simulink model "simulink_model"  (R2025b)
settings: Solver=VariableStepAuto  StartTime=0.0  StopTime=10  MaxStep=0.01  RelTol=1e-3
InitFcn:
  | addpath('C:\Users\prest\Documents\GitHub\NUSTARS\Roll-Control\Plotting');
  | % Define the directory containing the CSV files
  | data_dir = 'C:\Users\prest\Documents\GitHub\NUSTARS\Roll-Control\Plotting\Data';
  | addpath('C:\Users\prest\Documents\GitHub\NUSTARS\Roll-Control\Plotting');
  | 
  | % Get a list of all CSV files in the directory
  | csv_files = dir(fullfile(data_dir, '*.csv'));
  | 
  | for k = 1:length(csv_files)
  |     flight_csv = fullfile(data_dir, csv_files(k).name);
  |     ft_main_roll_only(flight_csv);
  | end
libraries: slpidlib x2
settings Model: Creator=maxhu  LastModifiedBy=prest

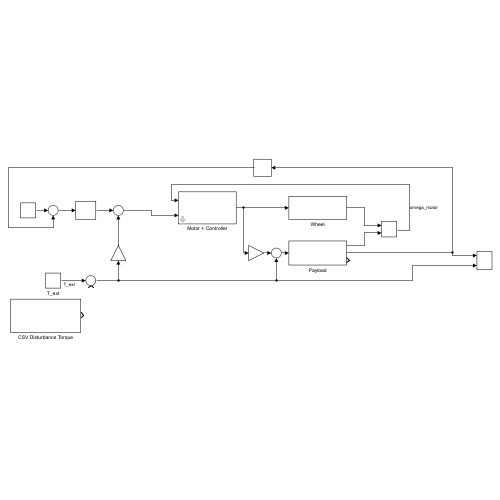
[thumbnail: Simulink's stored preview of the top-level diagram]
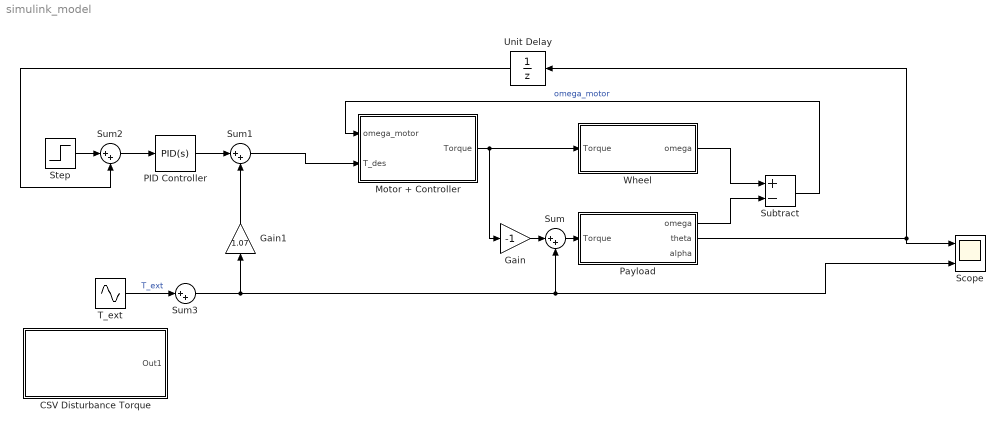
== system simulink_model ==
  CSV Disturbance Torque : Subsystem
  Gain : Gain  Gain=-1
  Gain1 : Gain  Gain=1.07
  Motor + Controller : Subsystem  mask{V_supply=12, T_max=1.65}
      mask prompts: V_supply "Battery Voltage [V]"; T_max "Max Torque [N*m]"
  PID Controller : slpidlib/PID Controller  Controller=PID  Form=Parallel  TimeDomain=Continuous-time  UseExternalTs=off  SampleTime=-1  IntegratorMethod=Forward Euler  FilterMethod=Forward Euler  ControllerParametersSource=internal  P=2e-1  I=5e-2  UseKiTs=off  D=8e-2  UseExternalDerivativeSource=off  N=30  UseFilter=on  TunerSelectOption=Transfer Function Based (PID Tuner App)  InitialConditionSource=internal  InitialConditionForIntegrator=0  InitialConditionForFilter=0  DifferentiatorICPrevScaledInput=0  ExternalReset=none  TrackingMode=off  Kt=1  LimitOutput=off  SatLimitsSource=internal  UpperSaturationLimit=inf  LowerSaturationLimit=-inf  LinearizeAsGain=on  AntiWindupMode=none  Kb=1  LimitIntegrator=on  UpperIntegratorSaturationLimit=1  LowerIntegratorSaturationLimit=-1  POutMin=[]  POutMax=[]  IOutMin=[]  IOutMax=[]  DOutMin=[]  DOutMax=[]  NOutMin=[]  NOutMax=[]  SumOutMin=[]  SumOutMax=[]  SaturationOutMin=[]  SaturationOutMax=[]  PParamMin=[]  PParamMax=[]  IParamMin=[]  IParamMax=[]  DParamMin=[]  DParamMax=[]  NParamMin=[]  NParamMax=[]  KbParamMin=[]  KbParamMax=[]  KtParamMin=[]  KtParamMax=[]  KbOutMin=[]  KbOutMax=[]  KtOutMin=[]  KtOutMax=[]  IntegratorOutMin=[]  IntegratorOutMax=[]  FilterOutMin=[]  FilterOutMax=[]  SumI1OutMin=[]  SumI1OutMax=[]  SumI2OutMin=[]  SumI2OutMax=[]  SumI3OutMin=[]  SumI3OutMax=[]  SumI4OutMin=[]  SumI4OutMax=[]  SumDOutMin=[]  SumDOutMax=[]  DifferentiatorOutMin=[]  DifferentiatorOutMax=[]  FilterDiffOutCoefMin=[]  FilterDiffOutCoefMax=[]  ReciprocalOutMin=[]  ReciprocalOutMax=[]  SumDenOutMin=[]  SumDenOutMax=[]  SumNumOutMin=[]  SumNumOutMax=[]  DivideOutMin=[]  DivideOutMax=[]  UdiffTsProdOutMin=[]  UdiffTsProdOutMax=[]  NTsProdOutMin=[]  NTsProdOutMax=[]  UintegralTsProdOutMin=[]  UintegralTsProdOutMax=[]  UngainTsProdOutMin=[]  UngainTsProdOutMax=[]  ClampingZeroOutDataTypeStr=Inherit: Inherit via back propagation  ClampingZeroOutMin=[]  ClampingZeroOutMax=[]  FilterDenConstantOutDataTypeStr=Inherit: Inherit via back propagation  FilterDenConstantOutMin=[]  FilterDenConstantOutMax=[]  PCopyOutDataTypeStr=Inherit: Inherit via back propagation  PCopyOutMin=[]  PCopyOutMax=[]  NCopyOutDataTypeStr=Inherit: Inherit via back propagation  NCopyOutMin=[]  NCopyOutMax=[]  IntegratorContinuousStateAttributes=''  IntegratorStateMustResolveToSignalObject=off  IntegratorRTWStateStorageClass=Auto  FilterContinuousStateAttributes=''  FilterStateMustResolveToSignalObject=off  FilterRTWStateStorageClass=Auto  ParallelPVariant=InternalParameters  IdealPVariant=Disabled  IVariant=InternalParameters  DVariant=InternalParameters  IntegratorVariant=Continuous  SatVariant=Disabled  AWVariant=Passthrough  PCopyVariant=Disabled  TRVariant=Disabled  FdbkBlocksVariant=Forward  IdealPFdbkVariant=Disabled  SatFdbkVariant=Disabled  DerivativeFilterVariant=ContFilter  NVariant=InternalParameters  NCopyVariant=Disabled  FilterICVariant=InternalICsFilter  IntegratorICVariant=InternalICs  ExternalResetVariant=Disabled  TRSumVariant=Passthrough  SumFdbkVariant=Disabled  SumVariant=Sum_PID  TsampFilterVariant=InternalTs  TsampNgainVariant=Passthrough  TsampIntegralVariant=Passthrough  ExternalSaturationOutDataTypeStr=Inherit: Same as second input  DerivativeSourceVariant=ErrorSignal  PreIntVariant=InternalPreInt
  Payload : Subsystem
  Scope : Scope  NumInputPorts=2
      settings: ActiveDisplayYMinimum=-2.4708061966220987  ActiveDisplayYMaximum=3.9877688102350177
  Step : Step  After=-1  SampleTime=0
  Subtract : Sum  Inputs=+-
  Sum{,1..3} (4 alike) : Sum  Inputs=|++
  T_ext : Sin  Frequency=7  SampleTime=0
  Unit Delay : UnitDelay  SampleTime=1e-3  HasFrameUpgradeWarning=on
  Wheel : Subsystem
  wires:
  Wheel/1(omega) -> Subtract/1
  Gain/1 -> Sum/1
  Sum/1 -> Payload/1(Torque)
  Payload/1(omega) -> Subtract/2
  Motor + Controller/1(Torque) -> Gain/1, Wheel/1(Torque)
  Subtract/1 -> Motor + Controller/1(omega_motor)  "omega_motor"
  Payload/2(theta) -> Scope/1, Unit Delay/1
  Step/1 -> Sum2/1
  Sum2/1 -> PID Controller/1
  Unit Delay/1 -> Sum2/2
  Sum1/1 -> Motor + Controller/2(T_des)
  Sum3/1 -> Scope/2, Sum/2, Gain1/1
  Gain1/1 -> Sum1/2
  PID Controller/1 -> Sum1/1
  T_ext/1 -> Sum3/1  "T_ext"

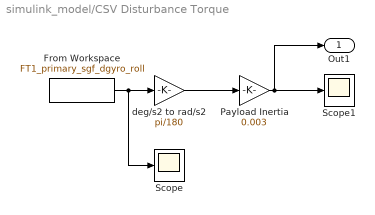
== system simulink_model/CSV Disturbance Torque ==
  From Workspace : FromWorkspace  VariableName=FT1_primary_sgf_dgyro_roll
  Payload Inertia : Gain  Gain=0.003
  Scope : Scope
      settings: ActiveDisplayYMinimum=-1  ActiveDisplayYMaximum=1  DataLoggingVariableName=ScopeData3
  Scope1 : Scope
      settings: ActiveDisplayYMinimum=-0.32143714141880175  ActiveDisplayYMaximum=0.6278113122409269
  deg/s2 to rad/s2 : Gain  Gain=pi/180
  Out1 : Outport
  wires:
  From Workspace/1 -> Scope/1, deg/s2 to rad/s2/1
  Payload Inertia/1 -> Out1/1, Scope1/1
  deg/s2 to rad/s2/1 -> Payload Inertia/1

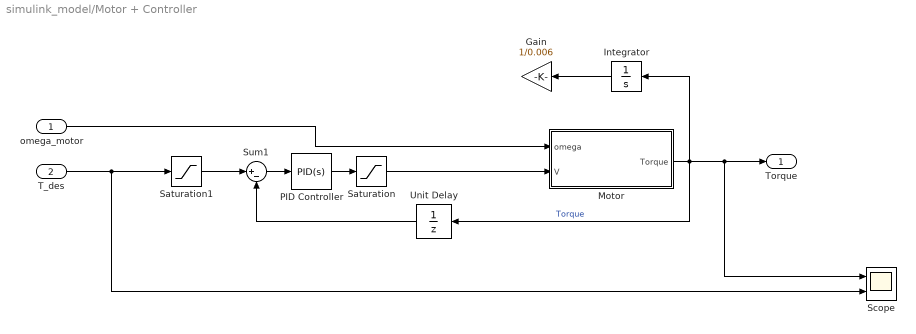
== system simulink_model/Motor + Controller ==
  omega_motor : Inport
  T_des : Inport  Port=2
  Gain : Gain  Gain=1/0.006
  Integrator : Integrator
  Motor : Subsystem  mask{w_nl=182, T_stall=10.9, L=0.000024}
      mask prompts: w_nl "No load speed [rad/s]"; T_stall "Stall torque [N*m]"; L "Inductance [H]"
  PID Controller : slpidlib/PID Controller  Controller=PID  Form=Parallel  TimeDomain=Continuous-time  UseExternalTs=off  SampleTime=-1  IntegratorMethod=Forward Euler  FilterMethod=Forward Euler  ControllerParametersSource=internal  P=1.24  I=650  UseKiTs=off  D=0.4e-4  UseExternalDerivativeSource=off  N=300  UseFilter=on  TunerSelectOption=Transfer Function Based (PID Tuner App)  InitialConditionSource=internal  InitialConditionForIntegrator=0  InitialConditionForFilter=0  DifferentiatorICPrevScaledInput=0  ExternalReset=none  TrackingMode=off  Kt=1  LimitOutput=on  SatLimitsSource=internal  UpperSaturationLimit=12  LowerSaturationLimit=-12  LinearizeAsGain=on  AntiWindupMode=none  Kb=1  LimitIntegrator=on  UpperIntegratorSaturationLimit=40  LowerIntegratorSaturationLimit=-40  POutMin=[]  POutMax=[]  IOutMin=[]  IOutMax=[]  DOutMin=[]  DOutMax=[]  NOutMin=[]  NOutMax=[]  SumOutMin=[]  SumOutMax=[]  SaturationOutMin=[]  SaturationOutMax=[]  PParamMin=[]  PParamMax=[]  IParamMin=[]  IParamMax=[]  DParamMin=[]  DParamMax=[]  NParamMin=[]  NParamMax=[]  KbParamMin=[]  KbParamMax=[]  KtParamMin=[]  KtParamMax=[]  KbOutMin=[]  KbOutMax=[]  KtOutMin=[]  KtOutMax=[]  IntegratorOutMin=[]  IntegratorOutMax=[]  FilterOutMin=[]  FilterOutMax=[]  SumI1OutMin=[]  SumI1OutMax=[]  SumI2OutMin=[]  SumI2OutMax=[]  SumI3OutMin=[]  SumI3OutMax=[]  SumI4OutMin=[]  SumI4OutMax=[]  SumDOutMin=[]  SumDOutMax=[]  DifferentiatorOutMin=[]  DifferentiatorOutMax=[]  FilterDiffOutCoefMin=[]  FilterDiffOutCoefMax=[]  ReciprocalOutMin=[]  ReciprocalOutMax=[]  SumDenOutMin=[]  SumDenOutMax=[]  SumNumOutMin=[]  SumNumOutMax=[]  DivideOutMin=[]  DivideOutMax=[]  UdiffTsProdOutMin=[]  UdiffTsProdOutMax=[]  NTsProdOutMin=[]  NTsProdOutMax=[]  UintegralTsProdOutMin=[]  UintegralTsProdOutMax=[]  UngainTsProdOutMin=[]  UngainTsProdOutMax=[]  ClampingZeroOutDataTypeStr=Inherit: Inherit via back propagation  ClampingZeroOutMin=[]  ClampingZeroOutMax=[]  FilterDenConstantOutDataTypeStr=Inherit: Inherit via back propagation  FilterDenConstantOutMin=[]  FilterDenConstantOutMax=[]  PCopyOutDataTypeStr=Inherit: Inherit via back propagation  PCopyOutMin=[]  PCopyOutMax=[]  NCopyOutDataTypeStr=Inherit: Inherit via back propagation  NCopyOutMin=[]  NCopyOutMax=[]  IntegratorContinuousStateAttributes=''  IntegratorStateMustResolveToSignalObject=off  IntegratorRTWStateStorageClass=Auto  FilterContinuousStateAttributes=''  FilterStateMustResolveToSignalObject=off  FilterRTWStateStorageClass=Auto  ParallelPVariant=InternalParameters  IdealPVariant=Disabled  IVariant=InternalParameters  DVariant=InternalParameters  IntegratorVariant=Continuous  SatVariant=Disabled  AWVariant=Passthrough  PCopyVariant=Disabled  TRVariant=Disabled  FdbkBlocksVariant=Forward  IdealPFdbkVariant=Disabled  SatFdbkVariant=Disabled  DerivativeFilterVariant=ContFilter  NVariant=InternalParameters  NCopyVariant=Disabled  FilterICVariant=InternalICsFilter  IntegratorICVariant=InternalICs  ExternalResetVariant=Disabled  TRSumVariant=Passthrough  SumFdbkVariant=Disabled  SumVariant=Sum_PID  TsampFilterVariant=InternalTs  TsampNgainVariant=Passthrough  TsampIntegralVariant=Passthrough  ExternalSaturationOutDataTypeStr=Inherit: Same as second input  DerivativeSourceVariant=ErrorSignal  PreIntVariant=InternalPreInt
  Saturation : Saturate  UpperLimit=V_supply  LowerLimit=-V_supply
  Saturation1 : Saturate  UpperLimit=T_max  LowerLimit=-T_max
  Scope : Scope  NumInputPorts=2
      settings: ActiveDisplayYMinimum=-1  ActiveDisplayYMaximum=1  DataLoggingVariableName=ScopeData2
  Sum1 : Sum  Inputs=|+-
  Unit Delay : UnitDelay  SampleTime=0.0005  HasFrameUpgradeWarning=on
  Torque : Outport
  wires:
  Sum1/1 -> PID Controller/1
  Unit Delay/1 -> Sum1/2
  Motor/1(Torque) -> Integrator/1, Unit Delay/1, Scope/1, Torque/1  "Torque"
  PID Controller/1 -> Saturation/1
  Integrator/1 -> Gain/1
  Saturation/1 -> Motor/2(V)
  Saturation1/1 -> Sum1/1
  T_des/1 -> Scope/2, Saturation1/1
  omega_motor/1 -> Motor/1(omega)

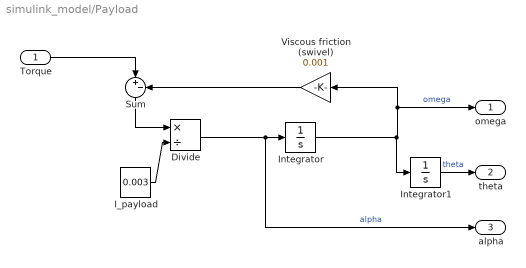
== system simulink_model/Payload ==
  Torque : Inport
  Divide : Product  Inputs=*/
  I_payload : Constant  Value=0.003
  Integrator : Integrator
  Integrator1 : Integrator
  Sum : Sum  Inputs=|+-
  Viscous friction (swivel) : Gain  Gain=0.001
  omega : Outport
  theta : Outport  Port=2
  alpha : Outport  Port=3
  wires:
  Integrator/1 -> Integrator1/1, Viscous friction (swivel)/1, omega/1  "omega"
  Sum/1 -> Divide/1
  Viscous friction (swivel)/1 -> Sum/2
  Torque/1 -> Sum/1
  I_payload/1 -> Divide/2
  Divide/1 -> alpha/1, Integrator/1  "alpha"
  Integrator1/1 -> theta/1  "theta"

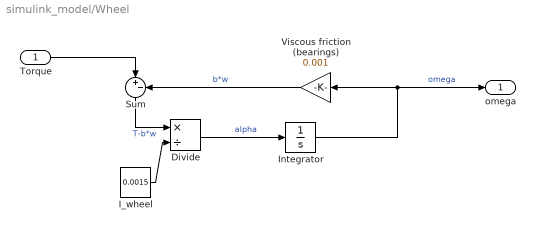
== system simulink_model/Wheel ==
  Torque : Inport
  Divide : Product  Inputs=*/
  I_wheel : Constant  Value=0.0015
  Integrator : Integrator
  Sum : Sum  Inputs=|+-
  Viscous friction (bearings) : Gain  Gain=0.001
  omega : Outport
  wires:
  Integrator/1 -> Viscous friction (bearings)/1, omega/1  "omega"
  Sum/1 -> Divide/1  "T-b*w"
  Torque/1 -> Sum/1
  I_wheel/1 -> Divide/2
  Divide/1 -> Integrator/1  "alpha"
  Viscous friction (bearings)/1 -> Sum/2  "b*w"

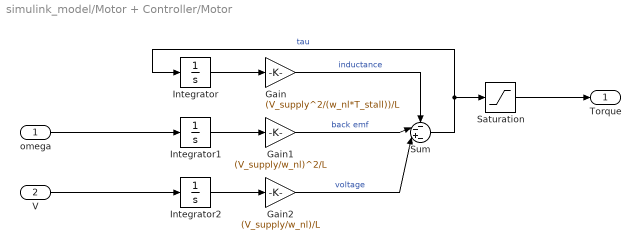
== system simulink_model/Motor + Controller/Motor ==
  omega : Inport
  V : Inport  Port=2
  Gain : Gain  Gain=(V_supply^2/(w_nl*T_stall))/L
  Gain1 : Gain  Gain=(V_supply/w_nl)^2/L
  Gain2 : Gain  Gain=(V_supply/w_nl)/L
  Integrator : Integrator
  Integrator1 : Integrator
  Integrator2 : Integrator
  Saturation : Saturate  UpperLimit=T_max  LowerLimit=-T_max
  Sum : Sum  Inputs=--+-
  Torque : Outport
  wires:
  Integrator/1 -> Gain/1
  Integrator1/1 -> Gain1/1
  Sum/1 -> Saturation/1, Integrator/1  "tau"
  Integrator2/1 -> Gain2/1
  Gain1/1 -> Sum/2  "back emf"
  Gain/1 -> Sum/1  "inductance"
  omega/1 -> Integrator1/1
  V/1 -> Integrator2/1
  Gain2/1 -> Sum/3  "voltage"
  Saturation/1 -> Torque/1
